simulink model "simuOp"  (R2024b)
settings: Solver=VariableStepAuto  StartTime=0.0  StopTime=10.0  RelTol=1e-3
values from neighbouring files (symbols this model uses):
  C1 = 1e-7    (= 1e-07)    [variables.m]
  C2 = 1e-7    (= 1e-07)    [variables.m]
  R1 = 5e+6    (= 5000000)    [variables.m]
  R2 = 5e+6    (= 5000000)    [variables.m]
  R3 = 5e+6    (= 5000000)    [variables.m]
settings Model: Creator=USER
settings RTWCC: GPUComputeCapability=3.5

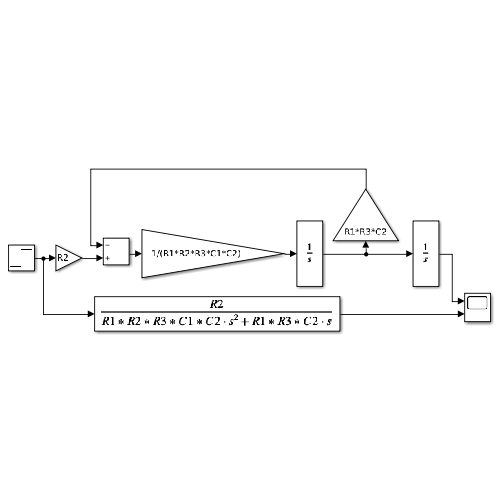
[thumbnail: Simulink's stored preview of the top-level diagram]
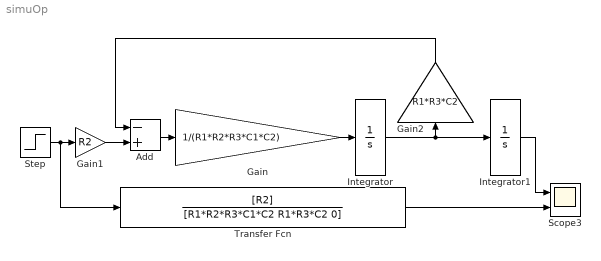
== system simuOp ==
  Add : Sum  Inputs=-+
  Gain : Gain  Gain=1/(R1*R2*R3*C1*C2)
  Gain1 : Gain  Gain=R2
  Gain2 : Gain  Gain=R1*R3*C2
  Integrator : Integrator
  Integrator1 : Integrator
  Scope3 : Scope  NumInputPorts=2
  Step : Step  Time=0  SampleTime=0
  Transfer Fcn : TransferFcn  Numerator=[R2]  Denominator=[R1*R2*R3*C1*C2 R1*R3*C2 0]
  wires:
  Integrator/1 -> Integrator1/1, Gain2/1
  Gain/1 -> Integrator/1
  Step/1 -> Transfer Fcn/1, Gain1/1
  Integrator1/1 -> Scope3/1
  Transfer Fcn/1 -> Scope3/2
  Gain2/1 -> Add/1
  Gain1/1 -> Add/2
  Add/1 -> Gain/1
